simulink model "Subsystem"  (R2020b)
settings: Solver=VariableStepAuto  StartTime=0.0  StopTime=10.0  RelTol=1e-3
settings Model: Creator=samar  LastModifiedBy=samar
settings DataIOCC: SaveOutput=off  SaveTime=off

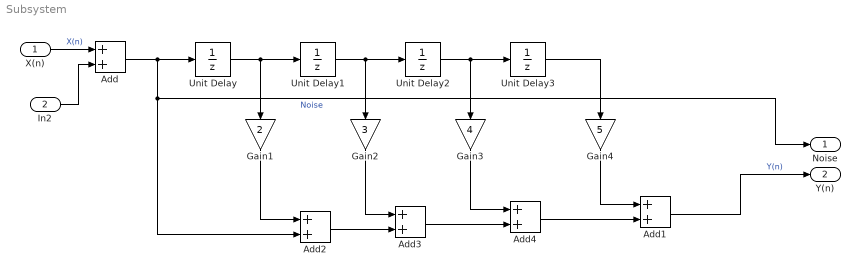
== system Subsystem ==
  X(n) : Inport  OutDataTypeStr=double  PortDimensions=1  SampleTime=0
  In2 : Inport  Port=2  OutDataTypeStr=double  PortDimensions=1  SampleTime=0
  Add{,1..4} (5 alike) : Sum
  Gain1 : Gain  Gain=2
  Gain2 : Gain  Gain=3
  Gain3 : Gain  Gain=4
  Gain4 : Gain  Gain=5
  Unit Delay{,1..3} (4 alike) : UnitDelay  SampleTime=-1  HasFrameUpgradeWarning=on
  Noise : Outport  OutDataTypeStr=double  PortDimensions=1  SampleTime=0
  Y(n) : Outport  Port=2  OutDataTypeStr=double  PortDimensions=1  SampleTime=0
  wires:
  Gain1/1 -> Add2/1
  Unit Delay1/1 -> Gain2/1, Unit Delay2/1
  X(n)/1 -> Add/1  "X(n)"
  Gain2/1 -> Add3/1
  Unit Delay2/1 -> Unit Delay3/1, Gain3/1
  Gain3/1 -> Add4/1
  Add4/1 -> Add1/2
  Unit Delay3/1 -> Gain4/1
  Add/1 -> Unit Delay/1, Add2/2, Noise/1  "Noise"
  Unit Delay/1 -> Gain1/1, Unit Delay1/1
  Add3/1 -> Add4/2
  Add2/1 -> Add3/2
  Gain4/1 -> Add1/1
  In2/1 -> Add/2
  Add1/1 -> Y(n)/1  "Y(n)"
